simulink model "wamjc7"  (Simulink 8.3)
settings: Solver=ode4  SolverMode=SingleTasking  StartTime=0.0  StopTime=inf  FixedStep=sample_time  RelTol=1e-3
undefined symbols (not defined in the file): arm_home, arm_home_norest, arm_j2mt, arm_m2jp, b, bit, C, CAN_init, enc_per_rev, FT_init, hand_on, MT_init, puck_I_per_Nm, rotFT2Hand, sample_time, Standard, VL1_init, VL2_init
libraries: xpclib x43, simulink x27, xpcutilitieslib x6, dspmathops x1, dspadpt3 x1, dspindex x1, dspbuff3 x1
(part 3 of 5)

== matlab function Subsystem/Plan Arm Trajectory/Compute qdes,qddes ==
  data: wdes output double; wddes output double; qdes_last input double; qddes_last input double; hand_on input double; sample_time input double; xdes input double; xddes input double; Tdes input double; pos input double; type input double; qdes output double; qddes output double; qdddes output double; q input double; error output double; FT input double
function [wdes,wddes,qdes,qddes,qdddes,error] = get_q(qdes_last,qddes_last,hand_on,sample_time,xdes,xddes,Tdes,pos,type,q,FT)
    % joint space move
    if(type == 0)
        qdes = xdes;
        qddes = xddes;
        qdddes = qddes - qddes_last;
        wdes = nan(7,1);
        wddes = nan(7,1);
        error = nan(6,1);
    % cartesian space move
    elseif (type == 1)
        % a, d, and alpha (b) DH parameters
        dh_a = [0 0 0.045 -0.045 0 0 0 0];
        dh_d = [0 0 0.55 0 0.3 0 .061 0]; % Not sure about dh_d(8) For the hand
        dh_b = [-pi/2 pi/2 -pi/2 pi/2 -pi/2 pi/2 0 0];
        
%         % Joint limits
%         qlim = [-2.62, 2.62; -2.01, 2.01; -2.97, 2.97; -0.87, 3.14; -4.79, 1.27; -1.57, 1.57; -3.0, 3.0;];
%         qmid = [0;0;0;1.135;1.76;0;0];  % The middle of the range for each joint

        % hand on
        if (hand_on)
            dh_d(8) = 0.0953; % Schunk Gripper
        end
        
        qFull = [q; 0];

        ct = cos(qFull);
        st = sin(qFull);
        cb = cos(dh_b);
        sb = sin(dh_b);

        % compute forward kinematics of current position
        T0 = eye(4);
        for i=1:8
            T = [ ct(i), -st(i)*cb(i),  st(i)*sb(i), dh_a(i)*ct(i);
                  st(i),  ct(i)*cb(i), -ct(i)*sb(i), dh_a(i)*st(i);
                  0, sb(i), cb(i), dh_d(i);
                  0, 0, 0, 1 ];
            T0 = T0*T;
        end
        
        % compute the tool configuration Jacobian (equation came from matlab symbolic math)
        % ct = cos(qdes_last);
        % st = sin(qdes_last);
        if hand_on
           % Jacobian for dh_d(8) = .0953  NEED TO RECOMPUTE JACOBIAN IF ANOTHER dh_d(8) IS USED
          V = [ (9*ct(4)*(ct(1)*st(3) + ct(2)*ct(3)*st(1)))/200 - (1563*st(6)*(st(5)*(ct(1)*ct(3) - ct(2)*st(1)*st(3)) + ct(5)*(ct(4)*(ct(1)*st(3) + ct(2)*ct(3)*st(1)) - st(1)*st(2)*st(4))))/10000 - (9*ct(1)*st(3))/200 - (11*st(1)*st(2))/20 - (1563*ct(6)*(st(4)*(ct(1)*st(3) + ct(2)*ct(3)*st(1)) + ct(4)*st(1)*st(2)))/10000 - (3*st(4)*(ct(1)*st(3) + ct(2)*ct(3)*st(1)))/10 - (9*ct(2)*ct(3)*st(1))/200 - (3*ct(4)*st(1)*st(2))/10 - (9*st(1)*st(2)*st(4))/200, (11*ct(1)*ct(2))/20 - (1563*st(6)*(ct(5)*(ct(1)*ct(2)*st(4) + ct(1)*ct(3)*ct(4)*st(2)) - ct(1)*st(2)*st(3)*st(5)))/10000 + (1563*ct(6)*(ct(1)*ct(2)*ct(4) - ct(1)*ct(3)*st(2)*st(4)))/10000 + (3*ct(1)*ct(2)*ct(4))/10 - (9*ct(1)*ct(3)*st(2))/200 + (9*ct(1)*ct(2)*st(4))/200 - (3*ct(1)*ct(3)*st(2)*st(4))/10 + (9*ct(1)*ct(3)*ct(4)*st(2))/200, (1563*st(6)*(st(5)*(st(1)*st(3) - ct(1)*ct(2)*ct(3)) - ct(4)*ct(5)*(ct(3)*st(1) + ct(1)*ct(2)*st(3))))/10000 - (9*ct(3)*st(1))/200 - (3*st(4)*(ct(3)*st(1) + ct(1)*ct(2)*st(3)))/10 + (9*ct(4)*(ct(3)*st(1) + ct(1)*ct(2)*st(3)))/200 - (1563*ct(6)*st(4)*(ct(3)*st(1) + ct(1)*ct(2)*st(3)))/10000 - (9*ct(1)*ct(2)*st(3))/200, (1563*ct(5)*st(6)*(st(4)*(st(1)*st(3) - ct(1)*ct(2)*ct(3)) - ct(1)*ct(4)*st(2)))/10000 - (1563*ct(6)*(ct(4)*(st(1)*st(3) - ct(1)*ct(2)*ct(3)) + ct(1)*st(2)*st(4)))/10000 - (3*ct(4)*(st(1)*st(3) - ct(1)*ct(2)*ct(3)))/10 - (9*st(4)*(st(1)*st(3) - ct(1)*ct(2)*ct(3)))/200 + (9*ct(1)*ct(4)*st(2))/200 - (3*ct(1)*st(2)*st(4))/10,  (1563*st(6)*(st(5)*(ct(4)*(st(1)*st(3) - ct(1)*ct(2)*ct(3)) + ct(1)*st(2)*st(4)) - ct(5)*(ct(3)*st(1) + ct(1)*ct(2)*st(3))))/10000, (1563*st(6)*(st(4)*(st(1)*st(3) - ct(1)*ct(2)*ct(3)) - ct(1)*ct(4)*st(2)))/10000 - (1563*ct(6)*(st(5)*(ct(3)*st(1) + ct(1)*ct(2)*st(3)) + ct(5)*(ct(4)*(st(1)*st(3) - ct(1)*ct(2)*ct(3)) + ct(1)*st(2)*st(4))))/10000,                                                                                                                                                                                             0;
                (11*ct(1)*st(2))/20 - (3*st(4)*(st(1)*st(3) - ct(1)*ct(2)*ct(3)))/10 - (9*st(1)*st(3))/200 - (1563*ct(6)*(st(4)*(st(1)*st(3) - ct(1)*ct(2)*ct(3)) - ct(1)*ct(4)*st(2)))/10000 + (9*ct(4)*(st(1)*st(3) - ct(1)*ct(2)*ct(3)))/200 - (1563*st(6)*(st(5)*(ct(3)*st(1) + ct(1)*ct(2)*st(3)) + ct(5)*(ct(4)*(st(1)*st(3) - ct(1)*ct(2)*ct(3)) + ct(1)*st(2)*st(4))))/10000 + (9*ct(1)*ct(2)*ct(3))/200 + (3*ct(1)*ct(4)*st(2))/10 + (9*ct(1)*st(2)*st(4))/200, (11*ct(2)*st(1))/20 - (1563*st(6)*(ct(5)*(ct(2)*st(1)*st(4) + ct(3)*ct(4)*st(1)*st(2)) - st(1)*st(2)*st(3)*st(5)))/10000 + (1563*ct(6)*(ct(2)*ct(4)*st(1) - ct(3)*st(1)*st(2)*st(4)))/10000 + (3*ct(2)*ct(4)*st(1))/10 - (9*ct(3)*st(1)*st(2))/200 + (9*ct(2)*st(1)*st(4))/200 + (9*ct(3)*ct(4)*st(1)*st(2))/200 - (3*ct(3)*st(1)*st(2)*st(4))/10, (3*st(4)*(ct(1)*ct(3) - ct(2)*st(1)*st(3)))/10 + (9*ct(1)*ct(3))/200 - (1563*st(6)*(st(5)*(ct(1)*st(3) + ct(2)*ct(3)*st(1)) - ct(4)*ct(5)*(ct(1)*ct(3) - ct(2)*st(1)*st(3))))/10000 - (9*ct(4)*(ct(1)*ct(3) - ct(2)*st(1)*st(3)))/200 + (1563*ct(6)*st(4)*(ct(1)*ct(3) - ct(2)*st(1)*st(3)))/10000 - (9*ct(2)*st(1)*st(3))/200, (9*st(4)*(ct(1)*st(3) + ct(2)*ct(3)*st(1)))/200 + (1563*ct(6)*(ct(4)*(ct(1)*st(3) + ct(2)*ct(3)*st(1)) - st(1)*st(2)*st(4)))/10000 + (3*ct(4)*(ct(1)*st(3) + ct(2)*ct(3)*st(1)))/10 - (1563*ct(5)*st(6)*(st(4)*(ct(1)*st(3) + ct(2)*ct(3)*st(1)) + ct(4)*st(1)*st(2)))/10000 + (9*ct(4)*st(1)*st(2))/200 - (3*st(1)*st(2)*st(4))/10, -(1563*st(6)*(st(5)*(ct(4)*(ct(1)*st(3) + ct(2)*ct(3)*st(1)) - st(1)*st(2)*st(4)) - ct(5)*(ct(1)*ct(3) - ct(2)*st(1)*st(3))))/10000, (1563*ct(6)*(st(5)*(ct(1)*ct(3) - ct(2)*st(1)*st(3)) + ct(5)*(ct(4)*(ct(1)*st(3) + ct(2)*ct(3)*st(1)) - st(1)*st(2)*st(4))))/10000 - (1563*st(6)*(st(4)*(ct(1)*st(3) + ct(2)*ct(3)*st(1)) + ct(4)*st(1)*st(2)))/10000,                                                                                                                                                                                             0;
                                                                                                                                                                                                                                                                                                                                                                                                                                                                      0,                                                                   (1563*st(6)*(ct(5)*(st(2)*st(4) - ct(2)*ct(3)*ct(4)) + ct(2)*st(3)*st(5)))/10000 - (9*ct(2)*ct(3))/200 - (3*ct(4)*st(2))/10 - (9*st(2)*st(4))/200 - (11*st(2))/20 - (1563*ct(6)*(ct(4)*st(2) + ct(2)*ct(3)*st(4)))/10000 + (9*ct(2)*ct(3)*ct(4))/200 - (3*ct(2)*ct(3)*st(4))/10,                                                                                                                                           (9*st(2)*st(3))/200 + (1563*st(6)*(ct(3)*st(2)*st(5) + ct(4)*ct(5)*st(2)*st(3)))/10000 - (9*ct(4)*st(2)*st(3))/200 + (3*st(2)*st(3)*st(4))/10 + (1563*ct(6)*st(2)*st(3)*st(4))/10000,                                                                                                                 (9*ct(2)*ct(4))/200 - (3*ct(2)*st(4))/10 - (1563*ct(6)*(ct(2)*st(4) + ct(3)*ct(4)*st(2)))/10000 - (1563*ct(5)*st(6)*(ct(2)*ct(4) - ct(3)*st(2)*st(4)))/10000 - (3*ct(3)*ct(4)*st(2))/10 - (9*ct(3)*st(2)*st(4))/200,                                                    (1563*st(6)*(st(5)*(ct(2)*st(4) + ct(3)*ct(4)*st(2)) + ct(5)*st(2)*st(3)))/10000,                                                                             - (1563*st(6)*(ct(2)*ct(4) - ct(3)*st(2)*st(4)))/10000 - (1563*ct(6)*(ct(5)*(ct(2)*st(4) + ct(3)*ct(4)*st(2)) - st(2)*st(3)*st(5)))/10000,                                                                                                                                                                                             0;
                                                                                                                                                                                                                                                                                                                                                                                                                                                                      0,                                                                                                                                                                                                                                                                                                                                            -st(1),                                                                                                                                                                                                                                                                                                                    ct(1)*st(2),                                                                                                                                                                                                                                                                                                   - ct(3)*st(1) - ct(1)*ct(2)*st(3),                                                                         ct(1)*ct(4)*st(2) - st(4)*(st(1)*st(3) - ct(1)*ct(2)*ct(3)),                                                                                                         st(5)*(ct(4)*(st(1)*st(3) - ct(1)*ct(2)*ct(3)) + ct(1)*st(2)*st(4)) - ct(5)*(ct(3)*st(1) + ct(1)*ct(2)*st(3)), - ct(6)*(st(4)*(st(1)*st(3) - ct(1)*ct(2)*ct(3)) - ct(1)*ct(4)*st(2)) - st(6)*(st(5)*(ct(3)*st(1) + ct(1)*ct(2)*st(3)) + ct(5)*(ct(4)*(st(1)*st(3) - ct(1)*ct(2)*ct(3)) + ct(1)*st(2)*st(4)));
                                                                                                                                                                                                                                                                                                                                                                                                                                                                      0,                                                                                                                                                                                                                                                                                                                                             ct(1),                                                                                                                                                                                                                                                                                                                    st(1)*st(2),                                                                                                                                                                                                                                                                                                     ct(1)*ct(3) - ct(2)*st(1)*st(3),                                                                         st(4)*(ct(1)*st(3) + ct(2)*ct(3)*st(1)) + ct(4)*st(1)*st(2),                                                                                                         ct(5)*(ct(1)*ct(3) - ct(2)*st(1)*st(3)) - st(5)*(ct(4)*(ct(1)*st(3) + ct(2)*ct(3)*st(1)) - st(1)*st(2)*st(4)),   st(6)*(st(5)*(ct(1)*ct(3) - ct(2)*st(1)*st(3)) + ct(5)*(ct(4)*(ct(1)*st(3) + ct(2)*ct(3)*st(1)) - st(1)*st(2)*st(4))) + ct(6)*(st(4)*(ct(1)*st(3) + ct(2)*ct(3)*st(1)) + ct(4)*st(1)*st(2));
                                                                                                                                                                                                                                                                                                                                                                                                                                                                      1,                                                                                                                                                                                                                                                                                                                                                 0,                                                                                                                                                                                                                                                                                                                          ct(2),                                                                                                                                                                                                                                                                                                                         st(2)*st(3),                                                                                                     ct(2)*ct(4) - ct(3)*st(2)*st(4),                                                                                                                                                           st(5)*(ct(2)*st(4) + ct(3)*ct(4)*st(2)) + ct(5)*st(2)*st(3),                                                                                 ct(6)*(ct(2)*ct(4) - ct(3)*st(2)*st(4)) - st(6)*(ct(5)*(ct(2)*st(4) + ct(3)*ct(4)*st(2)) - st(2)*st(3)*st(5));];

        else
            V = [(9*ct(4)*(ct(1)*st(3) + ct(2)*ct(3)*st(1)))/200 - (11*st(1)*st(2))/20 - (61*ct(6)*(st(4)*(ct(1)*st(3) + ct(2)*ct(3)*st(1)) + ct(4)*st(1)*st(2)))/1000 - (9*ct(1)*st(3))/200 - (61*st(6)*(ct(5)*(ct(4)*(ct(1)*st(3) + ct(2)*ct(3)*st(1)) - st(1)*st(2)*st(4)) + st(5)*(ct(1)*ct(3) - ct(2)*st(1)*st(3))))/1000 - (3*st(4)*(ct(1)*st(3) + ct(2)*ct(3)*st(1)))/10 - (3*ct(4)*st(1)*st(2))/10 - (9*st(1)*st(2)*st(4))/200 - (9*ct(2)*ct(3)*st(1))/200, (11*ct(1)*ct(2))/20 + (61*ct(6)*(ct(1)*ct(2)*ct(4) - ct(1)*ct(3)*st(2)*st(4)))/1000 - (61*st(6)*(ct(5)*(ct(1)*ct(2)*st(4) + ct(1)*ct(3)*ct(4)*st(2)) - ct(1)*st(2)*st(3)*st(5)))/1000 + (3*ct(1)*ct(2)*ct(4))/10 - (9*ct(1)*ct(3)*st(2))/200 + (9*ct(1)*ct(2)*st(4))/200 + (9*ct(1)*ct(3)*ct(4)*st(2))/200 - (3*ct(1)*ct(3)*st(2)*st(4))/10, (9*ct(4)*(ct(3)*st(1) + ct(1)*ct(2)*st(3)))/200 - (9*ct(3)*st(1))/200 - (3*st(4)*(ct(3)*st(1) + ct(1)*ct(2)*st(3)))/10 + (61*st(6)*(st(5)*(st(1)*st(3) - ct(1)*ct(2)*ct(3)) - ct(4)*ct(5)*(ct(3)*st(1) + ct(1)*ct(2)*st(3))))/1000 - (61*ct(6)*st(4)*(ct(3)*st(1) + ct(1)*ct(2)*st(3)))/1000 - (9*ct(1)*ct(2)*st(3))/200, (61*ct(5)*st(6)*(st(4)*(st(1)*st(3) - ct(1)*ct(2)*ct(3)) - ct(1)*ct(4)*st(2)))/1000 - (3*ct(4)*(st(1)*st(3) - ct(1)*ct(2)*ct(3)))/10 - (9*st(4)*(st(1)*st(3) - ct(1)*ct(2)*ct(3)))/200 - (3*ct(1)*st(2)*st(4))/10 - (61*ct(6)*(ct(4)*(st(1)*st(3) - ct(1)*ct(2)*ct(3)) + ct(1)*st(2)*st(4)))/1000 + (9*ct(1)*ct(4)*st(2))/200,   (61*st(6)*(st(5)*(ct(4)*(st(1)*st(3) - ct(1)*ct(2)*ct(3)) + ct(1)*st(2)*st(4)) - ct(5)*(ct(3)*st(1) + ct(1)*ct(2)*st(3))))/1000, (61*st(6)*(st(4)*(st(1)*st(3) - ct(1)*ct(2)*ct(3)) - ct(1)*ct(4)*st(2)))/1000 - (61*ct(6)*(ct(5)*(ct(4)*(st(1)*st(3) - ct(1)*ct(2)*ct(3)) + ct(1)*st(2)*st(4)) + st(5)*(ct(3)*st(1) + ct(1)*ct(2)*st(3))))/1000,                                                                                                                                                                                             0;
                 (11*ct(1)*st(2))/20 - (9*st(1)*st(3))/200 - (61*ct(6)*(st(4)*(st(1)*st(3) - ct(1)*ct(2)*ct(3)) - ct(1)*ct(4)*st(2)))/1000 - (61*st(6)*(ct(5)*(ct(4)*(st(1)*st(3) - ct(1)*ct(2)*ct(3)) + ct(1)*st(2)*st(4)) + st(5)*(ct(3)*st(1) + ct(1)*ct(2)*st(3))))/1000 + (9*ct(4)*(st(1)*st(3) - ct(1)*ct(2)*ct(3)))/200 - (3*st(4)*(st(1)*st(3) - ct(1)*ct(2)*ct(3)))/10 + (9*ct(1)*st(2)*st(4))/200 + (9*ct(1)*ct(2)*ct(3))/200 + (3*ct(1)*ct(4)*st(2))/10, (11*ct(2)*st(1))/20 - (61*st(6)*(ct(5)*(ct(2)*st(1)*st(4) + ct(3)*ct(4)*st(1)*st(2)) - st(1)*st(2)*st(3)*st(5)))/1000 + (61*ct(6)*(ct(2)*ct(4)*st(1) - ct(3)*st(1)*st(2)*st(4)))/1000 - (9*ct(3)*st(1)*st(2))/200 + (9*ct(2)*st(1)*st(4))/200 + (3*ct(2)*ct(4)*st(1))/10 + (9*ct(3)*ct(4)*st(1)*st(2))/200 - (3*ct(3)*st(1)*st(2)*st(4))/10, (9*ct(1)*ct(3))/200 - (9*ct(4)*(ct(1)*ct(3) - ct(2)*st(1)*st(3)))/200 + (3*st(4)*(ct(1)*ct(3) - ct(2)*st(1)*st(3)))/10 - (61*st(6)*(st(5)*(ct(1)*st(3) + ct(2)*ct(3)*st(1)) - ct(4)*ct(5)*(ct(1)*ct(3) - ct(2)*st(1)*st(3))))/1000 - (9*ct(2)*st(1)*st(3))/200 + (61*ct(6)*st(4)*(ct(1)*ct(3) - ct(2)*st(1)*st(3)))/1000, (61*ct(6)*(ct(4)*(ct(1)*st(3) + ct(2)*ct(3)*st(1)) - st(1)*st(2)*st(4)))/1000 + (3*ct(4)*(ct(1)*st(3) + ct(2)*ct(3)*st(1)))/10 + (9*st(4)*(ct(1)*st(3) + ct(2)*ct(3)*st(1)))/200 + (9*ct(4)*st(1)*st(2))/200 - (3*st(1)*st(2)*st(4))/10 - (61*ct(5)*st(6)*(st(4)*(ct(1)*st(3) + ct(2)*ct(3)*st(1)) + ct(4)*st(1)*st(2)))/1000,  -(61*st(6)*(st(5)*(ct(4)*(ct(1)*st(3) + ct(2)*ct(3)*st(1)) - st(1)*st(2)*st(4)) - ct(5)*(ct(1)*ct(3) - ct(2)*st(1)*st(3))))/1000, (61*ct(6)*(ct(5)*(ct(4)*(ct(1)*st(3) + ct(2)*ct(3)*st(1)) - st(1)*st(2)*st(4)) + st(5)*(ct(1)*ct(3) - ct(2)*st(1)*st(3))))/1000 - (61*st(6)*(st(4)*(ct(1)*st(3) + ct(2)*ct(3)*st(1)) + ct(4)*st(1)*st(2)))/1000,                                                                                                                                                                                             0;
                                                                                                                                                                                                                                                                                                                                                                                                                                                                 0,                                                                   61*st(6)*(ct(5)*(st(2)*st(4) - ct(2)*ct(3)*ct(4)) + (ct(2)*st(3)*st(5)))/1000 - (9*ct(2)*ct(3))/200 - (3*ct(4)*st(2))/10 - (9*st(2)*st(4))/200 - (11*st(2))/20 - (61*ct(6)*(ct(4)*st(2) + ct(2)*ct(3)*st(4)))/1000 + (9*ct(2)*ct(3)*ct(4))/200 - (3*ct(2)*ct(3)*st(4))/10,                                                                                                                                           (9*st(2)*st(3))/200 + (61*st(6)*(ct(3)*st(2)*st(5) + ct(4)*ct(5)*st(2)*st(3)))/1000 - (9*ct(4)*st(2)*st(3))/200 + (3*st(2)*st(3)*st(4))/10 + (61*ct(6)*st(2)*st(3)*st(4))/1000,                                                                                                                 (9*ct(2)*ct(4))/200 - (3*ct(2)*st(4))/10 - (61*ct(6)*(ct(2)*st(4) + ct(3)*ct(4)*st(2)))/1000 - (9*ct(3)*st(2)*st(4))/200 - (61*ct(5)*st(6)*(ct(2)*ct(4) - ct(3)*st(2)*st(4)))/1000 - (3*ct(3)*ct(4)*st(2))/10,                                                     (61*st(6)*(st(5)*(ct(2)*st(4) + ct(3)*ct(4)*st(2)) + ct(5)*st(2)*st(3)))/1000,                                                                             - (61*ct(6)*(ct(5)*(ct(2)*st(4) + ct(3)*ct(4)*st(2)) - st(2)*st(3)*st(5)))/1000 - (61*st(6)*(ct(2)*ct(4) - ct(3)*st(2)*st(4)))/1000,                                                                                                                                                                                             0;
                                                                                                                                                                                                                                                                                                                                                                                                                                                                 0,                                                                                                                                                                                                                                                                                                                                      -st(1),                                                                                                                                                                                                                                                                                                              ct(1)*st(2),                                                                                                                                                                                                                                                                                             - ct(3)*st(1) - ct(1)*ct(2)*st(3),                                                                       ct(1)*ct(4)*st(2) - st(4)*(st(1)*st(3) - ct(1)*ct(2)*ct(3)),                                                                                                   st(5)*(ct(4)*(st(1)*st(3) - ct(1)*ct(2)*ct(3)) + ct(1)*st(2)*st(4)) - ct(5)*(ct(3)*st(1) + ct(1)*ct(2)*st(3)), - ct(6)*(st(4)*(st(1)*st(3) - ct(1)*ct(2)*ct(3)) - ct(1)*ct(4)*st(2)) - st(6)*(ct(5)*(ct(4)*(st(1)*st(3) - ct(1)*ct(2)*ct(3)) + ct(1)*st(2)*st(4)) + st(5)*(ct(3)*st(1) + ct(1)*ct(2)*st(3)));
                                                                                                                                                                                                                                                                                                                                                                                                                                                                 0,                                                                                                                                                                                                                                                                                                                                       ct(1),                                                                                                                                                                                                                                                                                                              st(1)*st(2),                                                                                                                                                                                                                                                                                               ct(1)*ct(3) - ct(2)*st(1)*st(3),                                                                       st(4)*(ct(1)*st(3) + ct(2)*ct(3)*st(1)) + ct(4)*st(1)*st(2),                                                                                                   ct(5)*(ct(1)*ct(3) - ct(2)*st(1)*st(3)) - st(5)*(ct(4)*(ct(1)*st(3) + ct(2)*ct(3)*st(1)) - st(1)*st(2)*st(4)),   ct(6)*(st(4)*(ct(1)*st(3) + ct(2)*ct(3)*st(1)) + ct(4)*st(1)*st(2)) + st(6)*(ct(5)*(ct(4)*(ct(1)*st(3) + ct(2)*ct(3)*st(1)) - st(1)*st(2)*st(4)) + st(5)*(ct(1)*ct(3) - ct(2)*st(1)*st(3)));
                                                                                                                                                                                                                                                                                                                                                                                                                                                                 1,                                                                                                                                                                                                                                                                                                                                           0,                                                                                                                                                                                                                                                                                                                    ct(2),                                                                                                                                                                                                                                                                                                                   st(2)*st(3),                                                                                                   ct(2)*ct(4) - ct(3)*st(2)*st(4),                                                                                                                                                     st(5)*(ct(2)*st(4) + ct(3)*ct(4)*st(2)) + ct(5)*st(2)*st(3),                                                                               ct(6)*(ct(2)*ct(4) - ct(3)*st(2)*st(4)) - st(6)*(ct(5)*(ct(2)*st(4) + ct(3)*ct(4)*st(2)) - st(2)*st(3)*st(5)) ];
        end
        wdes = nan(7,1);
        wddes = nan(7,1);
        
        % Uncomment this line to generate error from current position (Option 3)
        Tdes(1:3,4) = T0(1:3,4) + 0.5*(Tdes(1:3,4) - T0(1:3,4));
        
        error = tr2delta(T0,Tdes);

%         % Find joint that is closest to limit
%         joint = 3; % Default to joint 3
%         eps = .5; % Set the boundary to switch to a joint (over joint 3)
%         for i = 1:7
%             lowDist = abs(qlim(i,1) - q(i));
%             highDist = abs(qlim(i,2) - q(i));
%             if lowDist < abs(eps)
%                 eps = lowDist;
%                 joint = i;
%             elseif highDist < abs(eps)
%                 eps = highDist;
%                 joint = i;
%             end
%         end
%         
%         % Get the nullspace of the jacobian
%         [A,B,C] = svd(V);
%         N = C(:,7);
%         
%         % Set the desired velocity of the null space to be the correct direction for that joint
%         qddesNs = zeros(7,1);
%         qddesNs(joint) = qmid(joint) - q(joint);
%         qp = (N*pinv(N)*qddesNs);
%         
%         n = norm(V*qp);  % Check for magnitude of change of end effector pose due to self motion
 
        %qddes = .1*pinv(V)*error + 200*qp;
        qddes = pinv(V)*error;
        %qddes = .5*V'*error;
        
        % Make sure none of the joint accelerations are too high.
        % The max value of .0008 was picked by hand through trial and error on the WAM
        qdddes = (qddes - qddes_last)/sample_time;
        if max(abs(qdddes)) > .5
            qdddes = (qdddes / max(abs(qdddes))) * .5;
            qddes = qddes_last + qdddes*sample_time;
        end

        % Normalize qddes so that no joint velocities are too high
        if max(qddes) > 0.5 
            qddes = (qddes / max(abs(qddes)) ) * 0.5;
        end

        % Up date the desired joint angles
        qdes = qdes_last + qddes*sample_time;
        
    % A trajectory move
    elseif(type == 2)
        wdes = nan(7,1);
        wddes = nan(7,1);
        error = zeros(6,1);
        
        % Unpack the desired joint angles
        qdes = Tdes(1:7)';
        % Calculate derivatives
        qddes = (qdes - qdes_last)/sample_time;
        qdddes = (qddes - qddes_last)/sample_time;
        %qdddes = zeros(7,1);
        
    % A compliant close
    elseif type == 3

        % The acutal current gripper width
        %gripperWidth = FT(8);  % Uncomment to use actual gripper width
        gripperWidth = pos(2);  % Uncomment to use predicted gripper width
        finger = pos(1);
        
        % Distance of the fingertip we are trying to hold still along the palm's Y axis
        fingerTipPosition = finger*gripperWidth/2;
        
        % a, d, and alpha (b) DH parameters from base to fingertip
        dh_a = [0 0 0.045 -0.045 0 0 0 0];
        dh_d = [0 0 0.55 0 0.3 0 .061 0];
        dh_b = [-pi/2 pi/2 -pi/2 pi/2 -pi/2 pi/2 0 0];
        
        % hand on
        if (hand_on)
            dh_d(8) = 0.0953; % Schunk Gripper
        end
        
        qFull = [q;0;0;0];

        ct = cos(qFull);
        st = sin(qFull);
        cb = cos(dh_b);
        sb = sin(dh_b);

        % compute forward kinematics of current position
        T0 = eye(4);
        for i=1:8
            T = [ ct(i), -st(i)*cb(i),  st(i)*sb(i), dh_a(i)*ct(i);
                  st(i),  ct(i)*cb(i), -ct(i)*sb(i), dh_a(i)*st(i);
                  0, sb(i), cb(i), dh_d(i);
                  0, 0, 0, 1 ];
            T0 = T0*T;
        end
        
        % Add the rotated vector from palm to fingertip
        T0(1:3,4) = T0(1:3,4) + T0(1:3,1:3)*[0;fingerTipPosition;.073];
        
        V = [ (9*ct(4)*(ct(1)*st(3) + ct(2)*ct(3)*st(1)))/200 - (2293*st(6)*(st(5)*(ct(1)*ct(3) - ct(2)*st(1)*st(3)) + ct(5)*(ct(4)*(ct(1)*st(3) + ct(2)*ct(3)*st(1)) - st(1)*st(2)*st(4))))/10000 - fingerTipPosition*(st(7)*(st(6)*(st(4)*(ct(1)*st(3) + ct(2)*ct(3)*st(1)) + ct(4)*st(1)*st(2)) - ct(6)*(st(5)*(ct(1)*ct(3) - ct(2)*st(1)*st(3)) + ct(5)*(ct(4)*(ct(1)*st(3) + ct(2)*ct(3)*st(1)) - st(1)*st(2)*st(4)))) - ct(7)*(st(5)*(ct(4)*(ct(1)*st(3) + ct(2)*ct(3)*st(1)) - st(1)*st(2)*st(4)) - ct(5)*(ct(1)*ct(3) - ct(2)*st(1)*st(3)))) - (9*ct(1)*st(3))/200 - (11*st(1)*st(2))/20 - (2293*ct(6)*(st(4)*(ct(1)*st(3) + ct(2)*ct(3)*st(1)) + ct(4)*st(1)*st(2)))/10000 - (3*st(4)*(ct(1)*st(3) + ct(2)*ct(3)*st(1)))/10 - (9*ct(2)*ct(3)*st(1))/200 - (3*ct(4)*st(1)*st(2))/10 - (9*st(1)*st(2)*st(4))/200, fingerTipPosition*(st(7)*(st(6)*(ct(1)*ct(2)*ct(4) - ct(1)*ct(3)*st(2)*st(4)) + ct(6)*(ct(5)*(ct(1)*ct(2)*st(4) + ct(1)*ct(3)*ct(4)*st(2)) - ct(1)*st(2)*st(3)*st(5))) + ct(7)*(st(5)*(ct(1)*ct(2)*st(4) + ct(1)*ct(3)*ct(4)*st(2)) + ct(1)*ct(5)*st(2)*st(3))) - (2293*st(6)*(ct(5)*(ct(1)*ct(2)*st(4) + ct(1)*ct(3)*ct(4)*st(2)) - ct(1)*st(2)*st(3)*st(5)))/10000 + (11*ct(1)*ct(2))/20 + (2293*ct(6)*(ct(1)*ct(2)*ct(4) - ct(1)*ct(3)*st(2)*st(4)))/10000 + (3*ct(1)*ct(2)*ct(4))/10 - (9*ct(1)*ct(3)*st(2))/200 + (9*ct(1)*ct(2)*st(4))/200 - (3*ct(1)*ct(3)*st(2)*st(4))/10 + (9*ct(1)*ct(3)*ct(4)*st(2))/200, (2293*st(6)*(st(5)*(st(1)*st(3) - ct(1)*ct(2)*ct(3)) - ct(4)*ct(5)*(ct(3)*st(1) + ct(1)*ct(2)*st(3))))/10000 - (9*ct(3)*st(1))/200 - (3*st(4)*(ct(3)*st(1) + ct(1)*ct(2)*st(3)))/10 - fingerTipPosition*(st(7)*(ct(6)*(st(5)*(st(1)*st(3) - ct(1)*ct(2)*ct(3)) - ct(4)*ct(5)*(ct(3)*st(1) + ct(1)*ct(2)*st(3))) + st(4)*st(6)*(ct(3)*st(1) + ct(1)*ct(2)*st(3))) - ct(7)*(ct(5)*(st(1)*st(3) - ct(1)*ct(2)*ct(3)) + ct(4)*st(5)*(ct(3)*st(1) + ct(1)*ct(2)*st(3)))) + (9*ct(4)*(ct(3)*st(1) + ct(1)*ct(2)*st(3)))/200 - (2293*ct(6)*st(4)*(ct(3)*st(1) + ct(1)*ct(2)*st(3)))/10000 - (9*ct(1)*ct(2)*st(3))/200, (2293*ct(5)*st(6)*(st(4)*(st(1)*st(3) - ct(1)*ct(2)*ct(3)) - ct(1)*ct(4)*st(2)))/10000 - fingerTipPosition*(st(7)*(st(6)*(ct(4)*(st(1)*st(3) - ct(1)*ct(2)*ct(3)) + ct(1)*st(2)*st(4)) + ct(5)*ct(6)*(st(4)*(st(1)*st(3) - ct(1)*ct(2)*ct(3)) - ct(1)*ct(4)*st(2))) + ct(7)*st(5)*(st(4)*(st(1)*st(3) - ct(1)*ct(2)*ct(3)) - ct(1)*ct(4)*st(2))) - (2293*ct(6)*(ct(4)*(st(1)*st(3) - ct(1)*ct(2)*ct(3)) + ct(1)*st(2)*st(4)))/10000 - (3*ct(4)*(st(1)*st(3) - ct(1)*ct(2)*ct(3)))/10 - (9*st(4)*(st(1)*st(3) - ct(1)*ct(2)*ct(3)))/200 + (9*ct(1)*ct(4)*st(2))/200 - (3*ct(1)*st(2)*st(4))/10,   fingerTipPosition*(ct(7)*(st(5)*(ct(3)*st(1) + ct(1)*ct(2)*st(3)) + ct(5)*(ct(4)*(st(1)*st(3) - ct(1)*ct(2)*ct(3)) + ct(1)*st(2)*st(4))) - ct(6)*st(7)*(st(5)*(ct(4)*(st(1)*st(3) - ct(1)*ct(2)*ct(3)) + ct(1)*st(2)*st(4)) - ct(5)*(ct(3)*st(1) + ct(1)*ct(2)*st(3)))) + (2293*st(6)*(st(5)*(ct(4)*(st(1)*st(3) - ct(1)*ct(2)*ct(3)) + ct(1)*st(2)*st(4)) - ct(5)*(ct(3)*st(1) + ct(1)*ct(2)*st(3))))/10000, (2293*st(6)*(st(4)*(st(1)*st(3) - ct(1)*ct(2)*ct(3)) - ct(1)*ct(4)*st(2)))/10000 - (2293*ct(6)*(st(5)*(ct(3)*st(1) + ct(1)*ct(2)*st(3)) + ct(5)*(ct(4)*(st(1)*st(3) - ct(1)*ct(2)*ct(3)) + ct(1)*st(2)*st(4))))/10000 - fingerTipPosition*st(7)*(ct(6)*(st(4)*(st(1)*st(3) - ct(1)*ct(2)*ct(3)) - ct(1)*ct(4)*st(2)) + st(6)*(st(5)*(ct(3)*st(1) + ct(1)*ct(2)*st(3)) + ct(5)*(ct(4)*(st(1)*st(3) - ct(1)*ct(2)*ct(3)) + ct(1)*st(2)*st(4)))), -fingerTipPosition*(ct(7)*(st(6)*(st(4)*(st(1)*st(3) - ct(1)*ct(2)*ct(3)) - ct(1)*ct(4)*st(2)) - ct(6)*(st(5)*(ct(3)*st(1) + ct(1)*ct(2)*st(3)) + ct(5)*(ct(4)*(st(1)*st(3) - ct(1)*ct(2)*ct(3)) + ct(1)*st(2)*st(4)))) + st(7)*(st(5)*(ct(4)*(st(1)*st(3) - ct(1)*ct(2)*ct(3)) + ct(1)*st(2)*st(4)) - ct(5)*(ct(3)*st(1) + ct(1)*ct(2)*st(3))));
              (11*ct(1)*st(2))/20 - (3*st(4)*(st(1)*st(3) - ct(1)*ct(2)*ct(3)))/10 - (9*st(1)*st(3))/200 - (2293*ct(6)*(st(4)*(st(1)*st(3) - ct(1)*ct(2)*ct(3)) - ct(1)*ct(4)*st(2)))/10000 + fingerTipPosition*(ct(7)*(st(5)*(ct(4)*(st(1)*st(3) - ct(1)*ct(2)*ct(3)) + ct(1)*st(2)*st(4)) - ct(5)*(ct(3)*st(1) + ct(1)*ct(2)*st(3))) - st(7)*(st(6)*(st(4)*(st(1)*st(3) - ct(1)*ct(2)*ct(3)) - ct(1)*ct(4)*st(2)) - ct(6)*(st(5)*(ct(3)*st(1) + ct(1)*ct(2)*st(3)) + ct(5)*(ct(4)*(st(1)*st(3) - ct(1)*ct(2)*ct(3)) + ct(1)*st(2)*st(4))))) + (9*ct(4)*(st(1)*st(3) - ct(1)*ct(2)*ct(3)))/200 - (2293*st(6)*(st(5)*(ct(3)*st(1) + ct(1)*ct(2)*st(3)) + ct(5)*(ct(4)*(st(1)*st(3) - ct(1)*ct(2)*ct(3)) + ct(1)*st(2)*st(4))))/10000 + (9*ct(1)*ct(2)*ct(3))/200 + (3*ct(1)*ct(4)*st(2))/10 + (9*ct(1)*st(2)*st(4))/200, (11*ct(2)*st(1))/20 - (2293*st(6)*(ct(5)*(ct(2)*st(1)*st(4) + ct(3)*ct(4)*st(1)*st(2)) - st(1)*st(2)*st(3)*st(5)))/10000 + fingerTipPosition*(ct(7)*(st(5)*(ct(2)*st(1)*st(4) + ct(3)*ct(4)*st(1)*st(2)) + ct(5)*st(1)*st(2)*st(3)) + st(7)*(ct(6)*(ct(5)*(ct(2)*st(1)*st(4) + ct(3)*ct(4)*st(1)*st(2)) - st(1)*st(2)*st(3)*st(5)) + st(6)*(ct(2)*ct(4)*st(1) - ct(3)*st(1)*st(2)*st(4)))) + (2293*ct(6)*(ct(2)*ct(4)*st(1) - ct(3)*st(1)*st(2)*st(4)))/10000 + (3*ct(2)*ct(4)*st(1))/10 - (9*ct(3)*st(1)*st(2))/200 + (9*ct(2)*st(1)*st(4))/200 + (9*ct(3)*ct(4)*st(1)*st(2))/200 - (3*ct(3)*st(1)*st(2)*st(4))/10, (3*st(4)*(ct(1)*ct(3) - ct(2)*st(1)*st(3)))/10 + (9*ct(1)*ct(3))/200 - (2293*st(6)*(st(5)*(ct(1)*st(3) + ct(2)*ct(3)*st(1)) - ct(4)*ct(5)*(ct(1)*ct(3) - ct(2)*st(1)*st(3))))/10000 + fingerTipPosition*(st(7)*(ct(6)*(st(5)*(ct(1)*st(3) + ct(2)*ct(3)*st(1)) - ct(4)*ct(5)*(ct(1)*ct(3) - ct(2)*st(1)*st(3))) + st(4)*st(6)*(ct(1)*ct(3) - ct(2)*st(1)*st(3))) - ct(7)*(ct(5)*(ct(1)*st(3) + ct(2)*ct(3)*st(1)) + ct(4)*st(5)*(ct(1)*ct(3) - ct(2)*st(1)*st(3)))) - (9*ct(4)*(ct(1)*ct(3) - ct(2)*st(1)*st(3)))/200 + (2293*ct(6)*st(4)*(ct(1)*ct(3) - ct(2)*st(1)*st(3)))/10000 - (9*ct(2)*st(1)*st(3))/200, (9*st(4)*(ct(1)*st(3) + ct(2)*ct(3)*st(1)))/200 + fingerTipPosition*(st(7)*(st(6)*(ct(4)*(ct(1)*st(3) + ct(2)*ct(3)*st(1)) - st(1)*st(2)*st(4)) + ct(5)*ct(6)*(st(4)*(ct(1)*st(3) + ct(2)*ct(3)*st(1)) + ct(4)*st(1)*st(2))) + ct(7)*st(5)*(st(4)*(ct(1)*st(3) + ct(2)*ct(3)*st(1)) + ct(4)*st(1)*st(2))) + (2293*ct(6)*(ct(4)*(ct(1)*st(3) + ct(2)*ct(3)*st(1)) - st(1)*st(2)*st(4)))/10000 + (3*ct(4)*(ct(1)*st(3) + ct(2)*ct(3)*st(1)))/10 - (2293*ct(5)*st(6)*(st(4)*(ct(1)*st(3) + ct(2)*ct(3)*st(1)) + ct(4)*st(1)*st(2)))/10000 + (9*ct(4)*st(1)*st(2))/200 - (3*st(1)*st(2)*st(4))/10, - (2293*st(6)*(st(5)*(ct(4)*(ct(1)*st(3) + ct(2)*ct(3)*st(1)) - st(1)*st(2)*st(4)) - ct(5)*(ct(1)*ct(3) - ct(2)*st(1)*st(3))))/10000 - fingerTipPosition*(ct(7)*(st(5)*(ct(1)*ct(3) - ct(2)*st(1)*st(3)) + ct(5)*(ct(4)*(ct(1)*st(3) + ct(2)*ct(3)*st(1)) - st(1)*st(2)*st(4))) - ct(6)*st(7)*(st(5)*(ct(4)*(ct(1)*st(3) + ct(2)*ct(3)*st(1)) - st(1)*st(2)*st(4)) - ct(5)*(ct(1)*ct(3) - ct(2)*st(1)*st(3)))), (2293*ct(6)*(st(5)*(ct(1)*ct(3) - ct(2)*st(1)*st(3)) + ct(5)*(ct(4)*(ct(1)*st(3) + ct(2)*ct(3)*st(1)) - st(1)*st(2)*st(4))))/10000 - (2293*st(6)*(st(4)*(ct(1)*st(3) + ct(2)*ct(3)*st(1)) + ct(4)*st(1)*st(2)))/10000 + fingerTipPosition*st(7)*(st(6)*(st(5)*(ct(1)*ct(3) - ct(2)*st(1)*st(3)) + ct(5)*(ct(4)*(ct(1)*st(3) + ct(2)*ct(3)*st(1)) - st(1)*st(2)*st(4))) + ct(6)*(st(4)*(ct(1)*st(3) + ct(2)*ct(3)*st(1)) + ct(4)*st(1)*st(2))),  fingerTipPosition*(st(7)*(st(5)*(ct(4)*(ct(1)*st(3) + ct(2)*ct(3)*st(1)) - st(1)*st(2)*st(4)) - ct(5)*(ct(1)*ct(3) - ct(2)*st(1)*st(3))) + ct(7)*(st(6)*(st(4)*(ct(1)*st(3) + ct(2)*ct(3)*st(1)) + ct(4)*st(1)*st(2)) - ct(6)*(st(5)*(ct(1)*ct(3) - ct(2)*st(1)*st(3)) + ct(5)*(ct(4)*(ct(1)*st(3) + ct(2)*ct(3)*st(1)) - st(1)*st(2)*st(4)))));
                                                                                                                                                                                                                                                                                                                                                                                                                                                                                                                                                                                                                                                                                                                                                                                                                      0,                                                                                                                   (2293*st(6)*(ct(5)*(st(2)*st(4) - ct(2)*ct(3)*ct(4)) + ct(2)*st(3)*st(5)))/10000 - (9*ct(2)*ct(3))/200 - (3*ct(4)*st(2))/10 - (9*st(2)*st(4))/200 - (11*st(2))/20 - fingerTipPosition*(ct(7)*(st(5)*(st(2)*st(4) - ct(2)*ct(3)*ct(4)) - ct(2)*ct(5)*st(3)) + st(7)*(st(6)*(ct(4)*st(2) + ct(2)*ct(3)*st(4)) + ct(6)*(ct(5)*(st(2)*st(4) - ct(2)*ct(3)*ct(4)) + ct(2)*st(3)*st(5)))) - (2293*ct(6)*(ct(4)*st(2) + ct(2)*ct(3)*st(4)))/10000 + (9*ct(2)*ct(3)*ct(4))/200 - (3*ct(2)*ct(3)*st(4))/10,                                                                                                                                                                                                                                                         (9*st(2)*st(3))/200 - fingerTipPosition*(st(7)*(ct(6)*(ct(3)*st(2)*st(5) + ct(4)*ct(5)*st(2)*st(3)) - st(2)*st(3)*st(4)*st(6)) - ct(7)*(ct(3)*ct(5)*st(2) - ct(4)*st(2)*st(3)*st(5))) + (2293*st(6)*(ct(3)*st(2)*st(5) + ct(4)*ct(5)*st(2)*st(3)))/10000 - (9*ct(4)*st(2)*st(3))/200 + (3*st(2)*st(3)*st(4))/10 + (2293*ct(6)*st(2)*st(3)*st(4))/10000,                                                                                                                                                                                                     (9*ct(2)*ct(4))/200 - fingerTipPosition*(st(7)*(st(6)*(ct(2)*st(4) + ct(3)*ct(4)*st(2)) - ct(5)*ct(6)*(ct(2)*ct(4) - ct(3)*st(2)*st(4))) - ct(7)*st(5)*(ct(2)*ct(4) - ct(3)*st(2)*st(4))) - (3*ct(2)*st(4))/10 - (2293*ct(6)*(ct(2)*st(4) + ct(3)*ct(4)*st(2)))/10000 - (2293*ct(5)*st(6)*(ct(2)*ct(4) - ct(3)*st(2)*st(4)))/10000 - (3*ct(3)*ct(4)*st(2))/10 - (9*ct(3)*st(2)*st(4))/200,                                                                                                                                                         fingerTipPosition*(ct(7)*(ct(5)*(ct(2)*st(4) + ct(3)*ct(4)*st(2)) - st(2)*st(3)*st(5)) - ct(6)*st(7)*(st(5)*(ct(2)*st(4) + ct(3)*ct(4)*st(2)) + ct(5)*st(2)*st(3))) + (2293*st(6)*(st(5)*(ct(2)*st(4) + ct(3)*ct(4)*st(2)) + ct(5)*st(2)*st(3)))/10000,                                                                                                                                                           - (2293*st(6)*(ct(2)*ct(4) - ct(3)*st(2)*st(4)))/10000 - (2293*ct(6)*(ct(5)*(ct(2)*st(4) + ct(3)*ct(4)*st(2)) - st(2)*st(3)*st(5)))/10000 - fingerTipPosition*st(7)*(st(6)*(ct(5)*(ct(2)*st(4) + ct(3)*ct(4)*st(2)) - st(2)*st(3)*st(5)) - ct(6)*(ct(2)*ct(4) - ct(3)*st(2)*st(4))),                                                                                                                                 -fingerTipPosition*(st(7)*(st(5)*(ct(2)*st(4) + ct(3)*ct(4)*st(2)) + ct(5)*st(2)*st(3)) - ct(7)*(st(6)*(ct(2)*ct(4) - ct(3)*st(2)*st(4)) + ct(6)*(ct(5)*(ct(2)*st(4) + ct(3)*ct(4)*st(2)) - st(2)*st(3)*st(5))));
                                                                                                                                                                                                                                                                                                                                                                                                                                                                                                                                                                                                                                                                                                                                                                                                                      0,                                                                                                                                                                                                                                                                                                                                                                                                                                                                                                                                                                                                              -st(1),                                                                                                                                                                                                                                                                                                                                                                                                                                                                                                                                                                                                    ct(1)*st(2),                                                                                                                                                                                                                                                                                                                                                                                                                                                                                                                                                             - ct(3)*st(1) - ct(1)*ct(2)*st(3),                                                                                                                                                                                                                                                                                                                                                    ct(1)*ct(4)*st(2) - st(4)*(st(1)*st(3) - ct(1)*ct(2)*ct(3)),                                                                                                                                                                                                                                                                                                                                 st(5)*(ct(4)*(st(1)*st(3) - ct(1)*ct(2)*ct(3)) + ct(1)*st(2)*st(4)) - ct(5)*(ct(3)*st(1) + ct(1)*ct(2)*st(3)),                                                                                                                                                    - ct(6)*(st(4)*(st(1)*st(3) - ct(1)*ct(2)*ct(3)) - ct(1)*ct(4)*st(2)) - st(6)*(st(5)*(ct(3)*st(1) + ct(1)*ct(2)*st(3)) + ct(5)*(ct(4)*(st(1)*st(3) - ct(1)*ct(2)*ct(3)) + ct(1)*st(2)*st(4)));
                                                                                                                                                                                                                                                                                                                                                                                                                                                                                                                                                                                                                                                                                                                                                                                                                      0,                                                                                                                                                                                                                                                                                                                                                                                                                                                                                                                                                                                                               ct(1),                                                                                                                                                                                                                                                                                                                                                                                                                                                                                                                                                                                                    st(1)*st(2),                                                                                                                                                                                                                                                                                                                                                                                                                                                                                                                                                               ct(1)*ct(3) - ct(2)*st(1)*st(3),                                                                                                                                                                                                                                                                                                                                                    st(4)*(ct(1)*st(3) + ct(2)*ct(3)*st(1)) + ct(4)*st(1)*st(2),                                                                                                                                                                                                                                                                                                                                 ct(5)*(ct(1)*ct(3) - ct(2)*st(1)*st(3)) - st(5)*(ct(4)*(ct(1)*st(3) + ct(2)*ct(3)*st(1)) - st(1)*st(2)*st(4)),                                                                                                                                                      st(6)*(st(5)*(ct(1)*ct(3) - ct(2)*st(1)*st(3)) + ct(5)*(ct(4)*(ct(1)*st(3) + ct(2)*ct(3)*st(1)) - st(1)*st(2)*st(4))) + ct(6)*(st(4)*(ct(1)*st(3) + ct(2)*ct(3)*st(1)) + ct(4)*st(1)*st(2));
                                                                                                                                                                                                                                                                                                                                                                                                                                                                                                                                                                                                                                                                                                                                                                                                                      1,                                                                                                                                                                                                                                                                                                                                                                                                                                                                                                                                                                                                                   0,                                                                                                                                                                                                                                                                                                                                                                                                                                                                                                                                                                                                          ct(2),                                                                                                                                                                                                                                                                                                                                                                                                                                                                                                                                                                                   st(2)*st(3),                                                                                                                                                                                                                                                                                                                                                                                ct(2)*ct(4) - ct(3)*st(2)*st(4),                                                                                                                                                                                                                                                                                                                                                                                   st(5)*(ct(2)*st(4) + ct(3)*ct(4)*st(2)) + ct(5)*st(2)*st(3),                                                                                                                                                                                                                                    ct(6)*(ct(2)*ct(4) - ct(3)*st(2)*st(4)) - st(6)*(ct(5)*(ct(2)*st(4) + ct(3)*ct(4)*st(2)) - st(2)*st(3)*st(5))];
        
        wdes = nan(7,1);
        wddes = nan(7,1);

        % Uncomment this line to generate error from current position (Option 3)
        %Tdes(1:3,4) = T0(1:3,4) + 0.5*(Tdes(1:3,4) - T0(1:3,4));

        error = tr2delta(T0,Tdes);
        
        %qddes = .1*pinv(V)*error + 200*qp;
        qddes = 10*pinv(V)*error;
        %qddes = .5*V'*error;
        
        % Make sure none of the joint accelerations are too high.
        % The max value of .5 was picked by hand through trial and error on the WAM
        qdddes = (qddes - qddes_last)/sample_time;
        if max(abs(qdddes)) > .5
            qdddes = (qdddes / max(abs(qdddes))) * .5;
            qddes = qddes_last + qdddes*sample_time;
        end

        % Normalize qddes so that no joint velocities are too high
        if max(qddes) > 0.5 
            qddes = (qddes / max(abs(qddes)) ) * 0.5;
        end

        % Up date the desired joint angles
        qdes = qdes_last + qddes*sample_time;
        
    elseif type == 5
        wdes = zeros(7,1);
        wddes = zeros(7,1);
        qdes = q;
        qddes = zeros(7,1);
        qdddes = zeros(7,1);
        error = zeros(6,1);
    else
        wdes = zeros(7,1);
        wddes = zeros(7,1);
        qdes = qdes_last;
        qddes = zeros(7,1);
        qdddes = zeros(7,1);
        error = zeros(6,1);
    end

end



%TR2DELTA Convert homogeneous transform to differential motion
%
% D = TR2DELTA(T0, T1) is the differential motion corresponding to 
% infinitessimal motion from pose T0 to T1 which are homogeneous 
% transformations. D=(dx, dy, dz, dRx, dRy, dRz) and is an approximation
% to the average spatial velocity multiplied by time.
%
% D = TR2DELTA(T) is the differential motion corresponding to the
% infinitessimal relative pose T expressed as a homogeneous 
% transformation.
%
% Notes::
% - D is only an approximation to the described by T, and assumes
%   that T0 ~ T1 or T ~ eye(4,4).
%
% See also DELTA2TR, SKEW.


% Copyright (C) 1993-2011, by Peter I. Corke
%
% This file is part of The Robotics Toolbox for Matlab (RTB).
% 
% RTB is free software: you can redistribute it and/or modify
% it under the terms of the GNU Lesser General Public License as published by
% the Free Software Foundation, either version 3 of the License, or
% (at your option) any later version.
% 
% RTB is distributed in the hope that it will be useful,
% but WITHOUT ANY WARRANTY; without even the implied warranty of
% MERCHANTABILITY or FITNESS FOR A PARTICULAR PURPOSE.  See the
% GNU Lesser General Public License for more details.
% 
% You should have received a copy of the GNU Leser General Public License
% along with RTB.  If not, see <http://www.gnu.org/licenses/>.

function delta = tr2delta(T0, T1)
    if nargin == 1
        T1 = T0;
        T0 = eye(4,4);
    end
    R0 = t2r(T0); R1 = t2r(T1);
    % in world frame
    delta = [ (T1(1:3,4)-T0(1:3,4)); vex( R1*R0' - eye(3,3)) ];
    % in T0 frame
    %delta = [ R0'*(T1(1:3,4)-T0(1:3,4)); R0'*vex( R1*R0' - eye(3,3)) ];

% TODO HACK understand/fix this and update Chapter 2
%    delta = [	T1(1:3,4)-T0(1:3,4);
%        0.5*(	cross(T0(1:3,1), T1(1:3,1)) + ...
%            cross(T0(1:3,2), T1(1:3,2)) + ...
%            cross(T0(1:3,3), T1(1:3,3)) ...
%        )];
end

%T2R Return rotational submatrix of a homogeneous transformation
%
% R = T2R(T) is the orthonormal rotation matrix component of homogeneous 
% transformation matrix T:
%
% Notes::
% - functions for T in SE(2) or SE(3)
%   - If T is 4x4, then R is 3x3.
%   - If T is 3x3, then R is  2x2.
% - the validity of rotational part is not checked
%
% See also R2T, TR2RT, RT2TR.


% Copyright (C) 1993-2011, by Peter I. Corke
%
% This file is part of The Robotics Toolbox for Matlab (RTB).
% 
% RTB is free software: you can redistribute it and/or modify
% it under the terms of the GNU Lesser General Public License as published by
% the Free Software Foundation, either version 3 of the License, or
% (at your option) any later version.
% 
% RTB is distributed in the hope that it will be useful,
% but WITHOUT ANY WARRANTY; without even the implied warranty of
% MERCHANTABILITY or FITNESS FOR A PARTICULAR PURPOSE.  See the
% GNU Lesser General Public License for more details.
% 
% You should have received a copy of the GNU Leser General Public License
% along with RTB.  If not, see <http://www.gnu.org/licenses/>.

function R = t2r(T)
    n = size(T,2);  % works for SE(2) or SE(3)
	R = T(1:n-1,1:n-1);
end

%VEX Convert skew-symmetric matrix to vector
%
% V = VEX(S) is the vector which has the skew-symmetric matrix S.
%
% Notes::
% - No checking is done to ensure that the matrix is skew-symmetric.
% - The function takes the mean of the two elements that correspond to each unique
%   element of the matrix, ie. vx = 0.5*(S(3,2)-S(2,3))
%
% See also SKEW.


% Copyright (C) 1993-2011, by Peter I. Corke
%
% This file is part of The Robotics Toolbox for Matlab (RTB).
% 
% RTB is free software: you can redistribute it and/or modify
% it under the terms of the GNU Lesser General Public License as published by
% the Free Software Foundation, either version 3 of the License, or
% (at your option) any later version.
% 
% RTB is distributed in the hope that it will be useful,
% but WITHOUT ANY WARRANTY; without even the implied warranty of
% MERCHANTABILITY or FITNESS FOR A PARTICULAR PURPOSE.  See the
% GNU Lesser General Public License for more details.
% 
% You should have received a copy of the GNU Leser General Public License
% along with RTB.  If not, see <http://www.gnu.org/licenses/>.

function v = vex(S)
    v = 0.5*[S(3,2)-S(2,3); S(1,3)-S(3,1); S(2,1)-S(1,2)];
end
